simulink model "simAttitudeControl"  (R2014b)
settings: Solver=ode45  StartTime=0.0  StopTime=tof  FixedStep=dt  MaxStep=dtmax  RelTol=1e-3
values from neighbouring files (symbols this model uses):
  dtFc = 10e-3    (= 0.01)    [quadrotor.m]
  euler0 = [0 0 0]'*pi/180    [quadrotor.m]
  IxxT = 2.7e-3    (= 0.0027)    [quadrotor.m]
  IyyT = IxxT    (= 0.0027)    [quadrotor.m]
  IzzT = 5.2e-3    (= 0.0052)    [quadrotor.m]
  Kp = 2*0.75*diag([1 1 1])    [quadrotor.m]
  Kv = 0*0.005*diag([1 1 1])    [quadrotor.m]
  pqr0 = [0 0 0]'*pi/180    [quadrotor.m]
  q0 = [euler0 ; pqr0]    [quadrotor.m]
  Vb0 = [0 0 0]'    [quadrotor.m]
  Xe0 = [0 0 0]'    [quadrotor.m]
libraries: aerolibutil x10
settings Model: Creator=alp.marangoz  LastModifiedBy=alpmarangoz
settings SolverCC: AutoInsertRateTranBlk=on
settings DataIOCC: SignalLoggingSaveFormat=ModelDataLogs
settings OptimizationCC: ExpressionDepthLimit=2147483647
settings DebuggingCC: UnderspecifiedInitializationDetection=Classic  MergeDetectMultiDrivingBlocksExec=none  InheritedTsInSrcMsg=none  CheckMatrixSingularityMsg=error  FcnCallInpInsideContextMsg=UseLocalSettings  StateNameClashWarn=warning
settings GRTTargetCC: CombineOutputUpdateFcns=off  GRTInterface=on

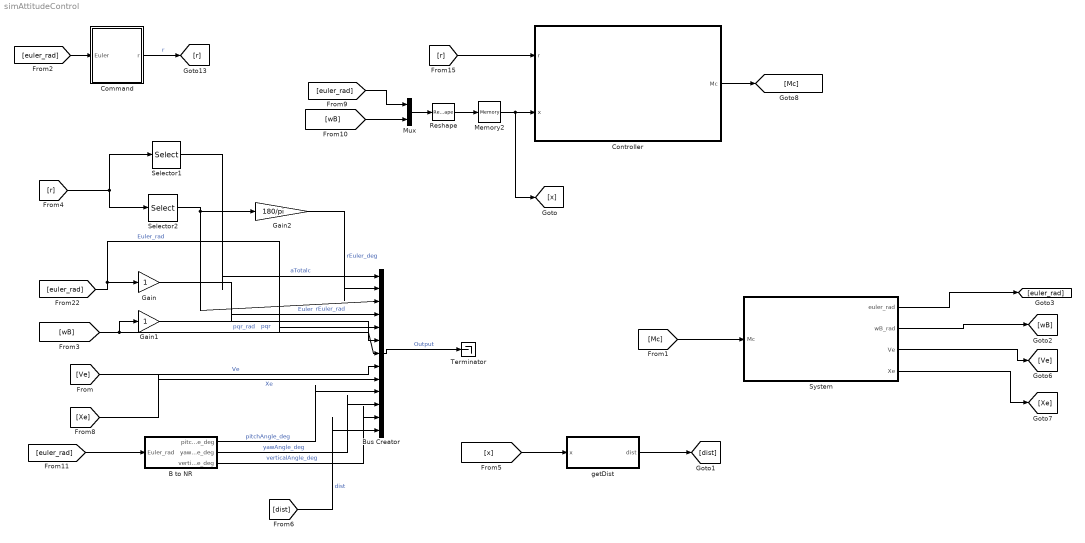
== system simAttitudeControl ==
  B to NR : Subsystem  TreatAsAtomicUnit=on
  Bus Creator : BusCreator  Inputs=13
  Command : Subsystem  TreatAsAtomicUnit=on  SystemSampleTime=dtFc
  Controller : Subsystem  TreatAsAtomicUnit=on  SystemSampleTime=dtFc
  Gain : Gain
  Gain1 : Gain
  Gain2 : Gain  Gain=180/pi
  Memory2 : Memory  X0=q0  InheritSampleTime=on  LinearizeMemory=on  LinearizeAsDelay=on
  Mux : Mux  Inputs=2
  Reshape : Reshape  OutputDimensionality=Column vector (2-D)
  Selector1 : Selector  NumberOfDimensions=2  InputPortWidth=2  IndexOptions=Index vector (dialog),Index vector (dialog)  Indices=1,1  OutputSizes=1,1
  Selector2 : Selector  NumberOfDimensions=2  InputPortWidth=3  IndexOptions=Index vector (dialog),Index vector (dialog)  Indices=[2 3 4],1  OutputSizes=1,1
  System : Subsystem  TreatAsAtomicUnit=on
  Terminator : Terminator
  getDist : Subsystem  TreatAsAtomicUnit=on
  wires:
  Command/1(r) -> [r]  "r"
  Controller/1(Mc) -> [Mc]
  [Mc] -> System/1(Mc)
  Reshape/1 -> Memory2/1
  [euler_rad] -> Command/1(Euler)
  Memory2/1 -> [x], Controller/2(x)
  [r] -> Controller/1(r)
  Bus Creator/1 -> Terminator/1  "Output"
  [r] -> Selector1/1, Selector2/1
  System/3(Ve) -> [Ve]
  System/4(Xe) -> [Xe]
  Selector1/1 -> Bus Creator/1  "aTotalc"
  Selector2/1 -> Gain2/1, Bus Creator/3  "rEuler_rad"
  [euler_rad] -> Gain/1, Bus Creator/5  "Euler_rad"
  [Ve] -> Bus Creator/8  "Ve"
  [Xe] -> Bus Creator/9  "Xe"
  System/1(euler_rad) -> [euler_rad]
  System/2(wB_rad) -> [wB]
  Mux/1 -> Reshape/1
  [euler_rad] -> Mux/1
  [wB] -> Mux/2
  Gain/1 -> Bus Creator/4  "Euler"
  [wB] -> Bus Creator/7, Gain1/1  "pqr_rad"
  Gain1/1 -> Bus Creator/6  "pqr"
  [euler_rad] -> B to NR/1(Euler_rad)
  B to NR/1(pitchAngle_deg) -> Bus Creator/10  "pitchAngle_deg"
  B to NR/2(yawAngle_deg) -> Bus Creator/11  "yawAngle_deg"
  B to NR/3(verticalAngle_deg) -> Bus Creator/12  "verticalAngle_deg"
  Gain2/1 -> Bus Creator/2  "rEuler_deg"
  [x] -> getDist/1(x)
  getDist/1(dist) -> [dist]
  [dist] -> Bus Creator/13  "dist"

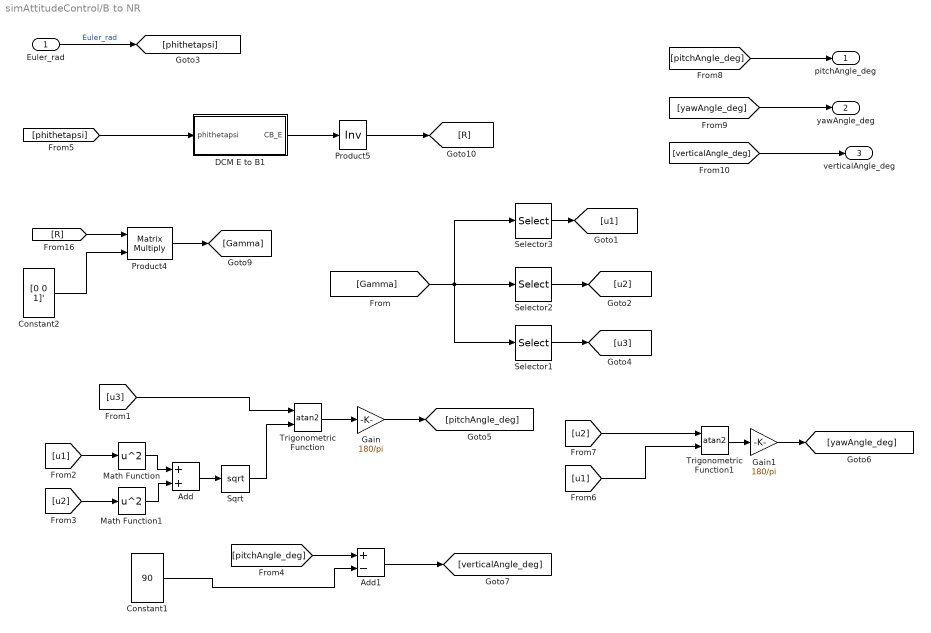
== system simAttitudeControl/B to NR ==
  Euler_rad : Inport
  Add : Sum
  Add1 : Sum  Inputs=+-
  Constant1 : Constant  Value=90  VectorParams1D=off
  Constant2 : Constant  Value=[0 0 1]'  VectorParams1D=off
  DCM E to B1 : Subsystem
  Gain : Gain  Gain=180/pi
  Gain1 : Gain  Gain=180/pi
  Math Function : Math  Operator=square  SaturateOnIntegerOverflow=on
  Math Function1 : Math  Operator=square  SaturateOnIntegerOverflow=on
  Product4 : Product  Multiplication=Matrix(*)  RndMeth=Zero
  Product5 : Product  Inputs=/  Multiplication=Matrix(*)  RndMeth=Zero
  Selector1 : Selector  InputPortWidth=3  Indices=3
  Selector2 : Selector  InputPortWidth=3  Indices=2
  Selector3 : Selector  InputPortWidth=3
  Sqrt : Sqrt  SaturateOnIntegerOverflow=on
  Trigonometric Function : Trigonometry  Operator=atan2
  Trigonometric Function1 : Trigonometry  Operator=atan2
  pitchAngle_deg : Outport
  yawAngle_deg : Outport  Port=2
  verticalAngle_deg : Outport  Port=3
  wires:
  Euler_rad/1 -> [phithetapsi]  "Euler_rad"
  Product5/1 -> [R]
  [phithetapsi] -> DCM E to B1/1(phithetapsi)
  DCM E to B1/1(CB_E) -> Product5/1
  [R] -> Product4/1
  Constant2/1 -> Product4/2
  Product4/1 -> [Gamma]
  [Gamma] -> Selector1/1, Selector3/1, Selector2/1
  Selector3/1 -> [u1]
  Selector2/1 -> [u2]
  Selector1/1 -> [u3]
  [u1] -> Math Function/1
  [u2] -> Math Function1/1
  Math Function/1 -> Add/1
  Math Function1/1 -> Add/2
  Add/1 -> Sqrt/1
  [u3] -> Trigonometric Function/1
  Sqrt/1 -> Trigonometric Function/2
  Trigonometric Function/1 -> Gain/1
  Trigonometric Function1/1 -> Gain1/1
  [u2] -> Trigonometric Function1/1
  [u1] -> Trigonometric Function1/2
  [yawAngle_deg] -> yawAngle_deg/1
  [pitchAngle_deg] -> pitchAngle_deg/1
  Gain/1 -> [pitchAngle_deg]
  Gain1/1 -> [yawAngle_deg]
  Constant1/1 -> Add1/2
  [pitchAngle_deg] -> Add1/1
  Add1/1 -> [verticalAngle_deg]
  [verticalAngle_deg] -> verticalAngle_deg/1

== system simAttitudeControl/Command ==
  Euler : Inport
  From Workspace : FromWorkspace  VariableName=r  Interpolate=off  OutputAfterFinalValue=Setting to zero
  Memory2 : Memory  X0=euler0  InheritSampleTime=on  LinearizeMemory=on  LinearizeAsDelay=on
  Reshape1 : Reshape  OutputDimensionality=Column vector (2-D)
  Selector : Selector  NumberOfDimensions=2  InputPortWidth=2  IndexOptions=Index vector (dialog),Index vector (dialog)  Indices=1,1  OutputSizes=1,1
  Selector1 : Selector  NumberOfDimensions=2  InputPortWidth=3  IndexOptions=Index vector (dialog),Index vector (dialog)  Indices=[2 3 4],1  OutputSizes=1,1
  Subtract : Sum  Inputs=+-
  Terminator : Terminator
  Terminator1 : Terminator
  Terminator2 : Terminator
  r : Outport  InitialOutput=0
  wires:
  From Workspace/1 -> Reshape1/1
  Reshape1/1 -> r/1, Selector/1, Selector1/1
  Euler/1 -> Memory2/1
  Memory2/1 -> [euler]
  [euler] -> Subtract/2  "q"
  Selector/1 -> Terminator/1  "rnc"
  Selector1/1 -> Terminator2/1, Subtract/1  "rEuler"
  Subtract/1 -> Terminator1/1  "eEuler"

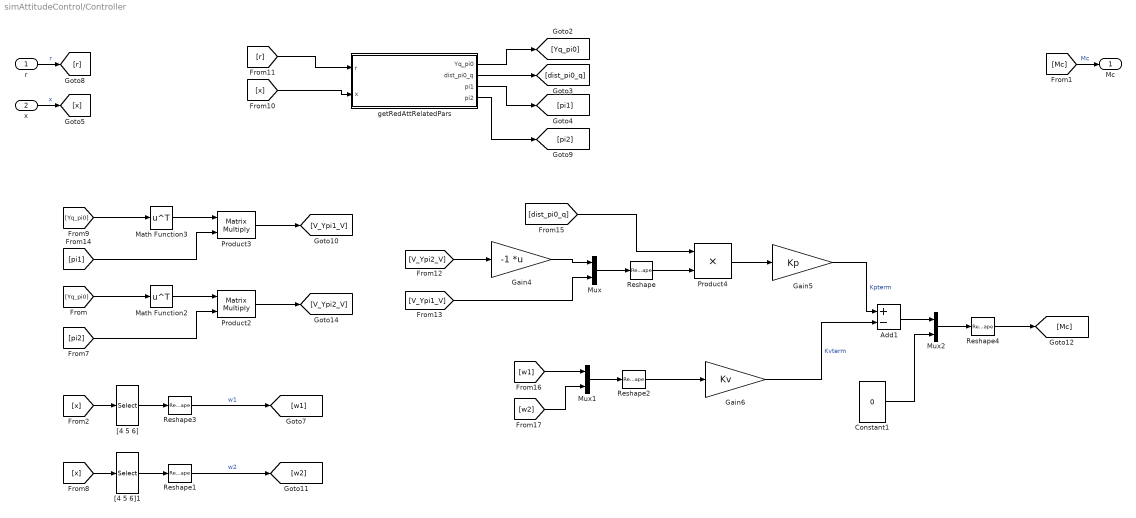
== system simAttitudeControl/Controller ==
  r : Inport
  x : Inport  Port=2
  Add1 : Sum  Inputs=+-
  Constant1 : Constant  Value=0  VectorParams1D=off
  Gain4 : Gain  Gain=-1  Multiplication=Matrix(K*u)
  Gain5 : Gain  Gain=Kp
  Gain6 : Gain  Gain=Kv
  Math Function2 : Math  Operator=transpose  SaturateOnIntegerOverflow=on
  Math Function3 : Math  Operator=transpose  SaturateOnIntegerOverflow=on
  Mux : Mux  Inputs=2
  Mux1 : Mux  Inputs=2
  Mux2 : Mux  Inputs=2
  Product2 : Product  Multiplication=Matrix(*)  RndMeth=Zero
  Product3 : Product  Multiplication=Matrix(*)  RndMeth=Zero
  Product4 : Product  RndMeth=Zero
  Reshape{,1..4} (5 alike) : Reshape  OutputDimensionality=Column vector (2-D)
  "[4 5 6]" : Selector  InputPortWidth=6  Indices=4
  "[4 5 6]1" : Selector  InputPortWidth=6  Indices=5
  getRedAttRelatedPars : Subsystem
  Mc : Outport
  wires:
  r/1 -> [r]  "r"
  x/1 -> [x]  "x"
  [Mc] -> Mc/1  "Mc"
  [x] -> getRedAttRelatedPars/2(x)
  [r] -> getRedAttRelatedPars/1(r)
  getRedAttRelatedPars/2(dist_pi0_q) -> [dist_pi0_q]
  getRedAttRelatedPars/1(Yq_pi0) -> [Yq_pi0]
  getRedAttRelatedPars/3(pi1) -> [pi1]
  getRedAttRelatedPars/4(pi2) -> [pi2]
  [Yq_pi0] -> Math Function2/1
  Math Function2/1 -> Product2/1
  [pi2] -> Product2/2
  Product2/1 -> [V_Ypi2_V]
  [Yq_pi0] -> Math Function3/1
  Math Function3/1 -> Product3/1
  [pi1] -> Product3/2
  Product3/1 -> [V_Ypi1_V]
  Reshape3/1 -> [w1]  "w1"
  "[4 5 6]"/1 -> Reshape3/1
  [x] -> "[4 5 6]"/1
  Reshape1/1 -> [w2]  "w2"
  "[4 5 6]1"/1 -> Reshape1/1
  [x] -> "[4 5 6]1"/1
  [V_Ypi2_V] -> Gain4/1
  Gain4/1 -> Mux/1
  [V_Ypi1_V] -> Mux/2
  Mux/1 -> Reshape/1
  [dist_pi0_q] -> Product4/1
  Reshape/1 -> Product4/2
  Product4/1 -> Gain5/1
  Mux1/1 -> Reshape2/1
  [w1] -> Mux1/1
  [w2] -> Mux1/2
  Reshape2/1 -> Gain6/1
  Gain5/1 -> Add1/1  "Kpterm"
  Gain6/1 -> Add1/2  "Kvterm"
  Mux2/1 -> Reshape4/1
  Add1/1 -> Mux2/1
  Constant1/1 -> Mux2/2
  Reshape4/1 -> [Mc]

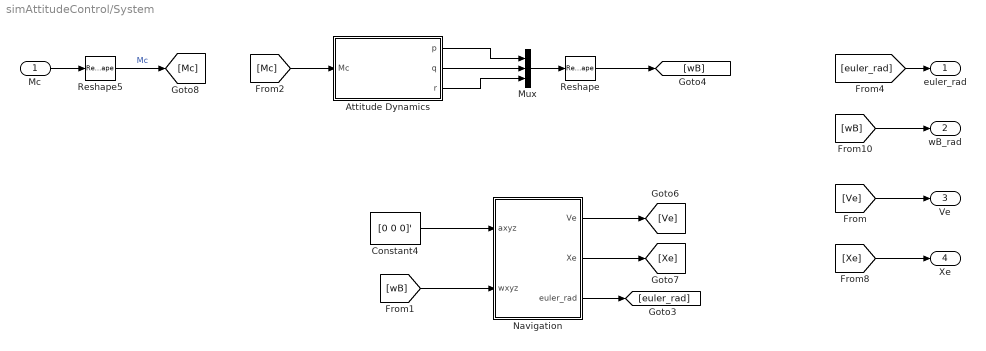
== system simAttitudeControl/System ==
  Mc : Inport
  Attitude Dynamics : Subsystem
  Constant4 : Constant  Value=[0 0 0]'  VectorParams1D=off
  Mux : Mux  Inputs=3
  Navigation : Subsystem
  Reshape : Reshape  OutputDimensionality=Column vector (2-D)
  Reshape5 : Reshape  OutputDimensionality=Column vector (2-D)
  euler_rad : Outport
  wB_rad : Outport  Port=2
  Ve : Outport  Port=3
  Xe : Outport  Port=4
  wires:
  Mc/1 -> Reshape5/1
  Reshape5/1 -> [Mc]  "Mc"
  [euler_rad] -> euler_rad/1
  Constant4/1 -> Navigation/1(axyz)
  [wB] -> Navigation/2(wxyz)
  Navigation/1(Ve) -> [Ve]
  Navigation/2(Xe) -> [Xe]
  Navigation/3(euler_rad) -> [euler_rad]
  [Xe] -> Xe/1
  [Ve] -> Ve/1
  [wB] -> wB_rad/1
  Attitude Dynamics/1(p) -> Mux/1
  Attitude Dynamics/2(q) -> Mux/2
  Attitude Dynamics/3(r) -> Mux/3
  Mux/1 -> Reshape/1
  Reshape/1 -> [wB]
  [Mc] -> Attitude Dynamics/1(Mc)

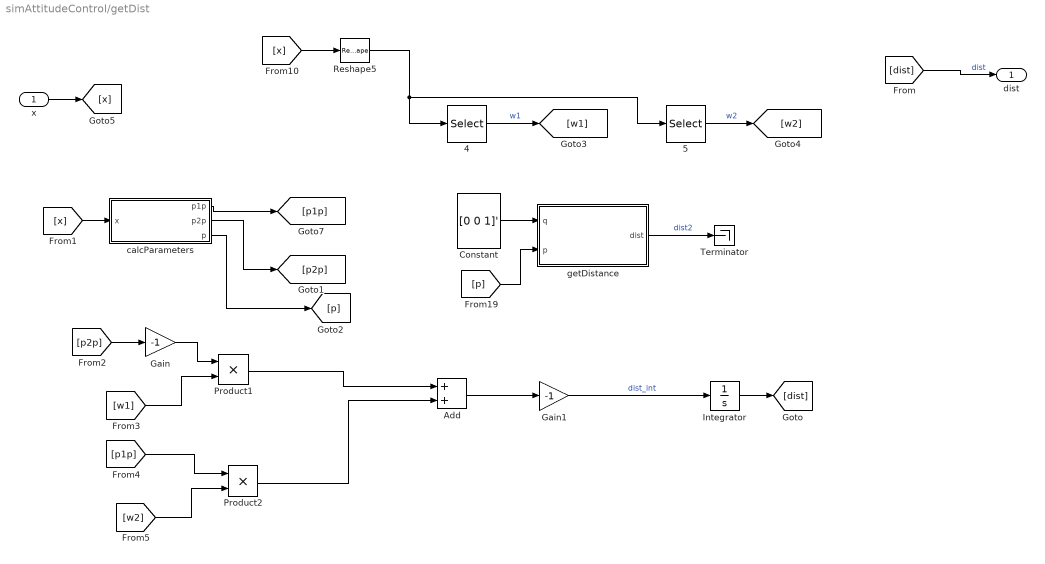
== system simAttitudeControl/getDist ==
  x : Inport
  4 : Selector  NumberOfDimensions=2  InputPortWidth=3  IndexOptions=Index vector (dialog),Index vector (dialog)  Indices=4,1  OutputSizes=1,1
  5 : Selector  NumberOfDimensions=2  InputPortWidth=3  IndexOptions=Index vector (dialog),Index vector (dialog)  Indices=5,1  OutputSizes=1,1
  Add : Sum
  Constant : Constant  Value=[0 0 1]'  VectorParams1D=off
  Gain : Gain  Gain=-1
  Gain1 : Gain  Gain=-1
  Integrator : Integrator
  Product1 : Product
  Product2 : Product
  Reshape5 : Reshape  OutputDimensionality=Column vector (2-D)
  Terminator : Terminator
  calcParameters : Subsystem  TreatAsAtomicUnit=on
  getDistance : Subsystem
  dist : Outport
  wires:
  x/1 -> [x]
  Reshape5/1 -> 5/1, 4/1
  [x] -> Reshape5/1
  [dist] -> dist/1  "dist"
  [x] -> calcParameters/1(x)
  calcParameters/1(p1p) -> [p1p]
  calcParameters/2(p2p) -> [p2p]
  4/1 -> [w1]  "w1"
  5/1 -> [w2]  "w2"
  [w1] -> Product1/2
  [p1p] -> Product2/1
  [w2] -> Product2/2
  [p2p] -> Gain/1
  Gain/1 -> Product1/1
  Product1/1 -> Add/1
  Product2/1 -> Add/2
  Add/1 -> Gain1/1
  Gain1/1 -> Integrator/1  "dist_int"
  Integrator/1 -> [dist]
  getDistance/1(dist) -> Terminator/1  "dist2"
  Constant/1 -> getDistance/1(q)
  [p] -> getDistance/2(p)
  calcParameters/3(p) -> [p]

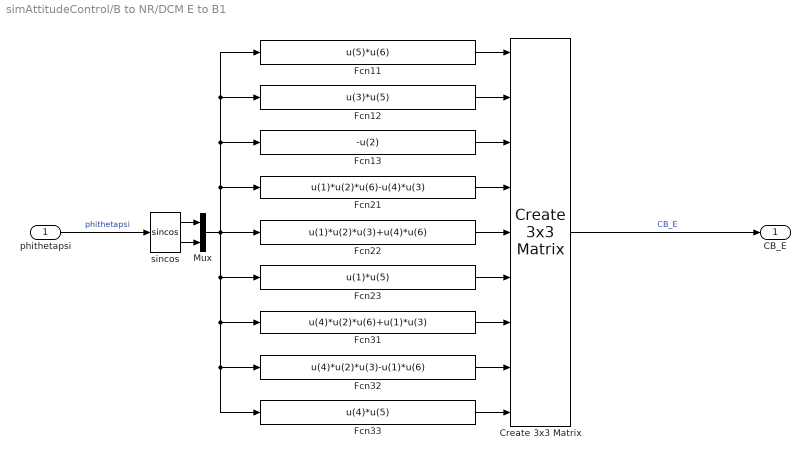
== system simAttitudeControl/B to NR/DCM E to B1 ==
  phithetapsi : Inport
  Create 3x3 Matrix : aerolibutil/Create 3x3 Matrix
  Fcn11 : Fcn  Expr=u(5)*u(6)
  Fcn12 : Fcn  Expr=u(3)*u(5)
  Fcn13 : Fcn  Expr=-u(2)
  Fcn21 : Fcn  Expr=u(1)*u(2)*u(6)-u(4)*u(3)
  Fcn22 : Fcn  Expr=u(1)*u(2)*u(3)+u(4)*u(6)
  Fcn23 : Fcn  Expr=u(1)*u(5)
  Fcn31 : Fcn  Expr=u(4)*u(2)*u(6)+u(1)*u(3)
  Fcn32 : Fcn  Expr=u(4)*u(2)*u(3)-u(1)*u(6)
  Fcn33 : Fcn  Expr=u(4)*u(5)
  Mux : Mux  Inputs=2
  sincos : Trigonometry  Operator=sincos
  CB_E : Outport
  wires:
  Create 3x3 Matrix/1 -> CB_E/1  "CB_E"
  phithetapsi/1 -> sincos/1  "phithetapsi"
  Fcn33/1 -> Create 3x3 Matrix/9
  Fcn32/1 -> Create 3x3 Matrix/8
  Fcn23/1 -> Create 3x3 Matrix/6
  Fcn22/1 -> Create 3x3 Matrix/5
  Fcn31/1 -> Create 3x3 Matrix/7
  Fcn21/1 -> Create 3x3 Matrix/4
  Fcn13/1 -> Create 3x3 Matrix/3
  Fcn12/1 -> Create 3x3 Matrix/2
  Fcn11/1 -> Create 3x3 Matrix/1
  Mux/1 -> Fcn21/1, Fcn13/1, Fcn12/1, Fcn11/1, Fcn22/1, Fcn23/1, Fcn31/1, Fcn33/1, Fcn32/1
  sincos/2 -> Mux/2
  sincos/1 -> Mux/1

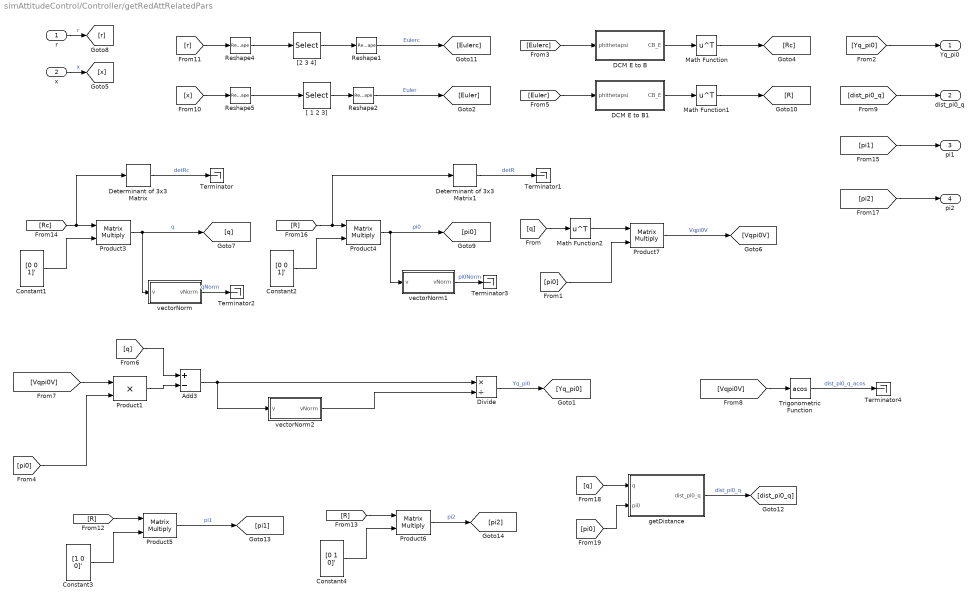
== system simAttitudeControl/Controller/getRedAttRelatedPars ==
  r : Inport
  x : Inport  Port=2
  Add3 : Sum  Inputs=+-
  Constant1 : Constant  Value=[0 0 1]'  VectorParams1D=off
  Constant2 : Constant  Value=[0 0 1]'  VectorParams1D=off
  Constant3 : Constant  Value=[1 0 0]'  VectorParams1D=off
  Constant4 : Constant  Value=[0 1 0]'  VectorParams1D=off
  DCM E to B : Subsystem
  DCM E to B1 : Subsystem
  Determinant of 3x3 Matrix : aerolibutil/Determinant of 3x3 Matrix
  Determinant of 3x3 Matrix1 : aerolibutil/Determinant of 3x3 Matrix
  Divide : Product  Inputs=*/
  Math Function : Math  Operator=transpose  SaturateOnIntegerOverflow=on
  Math Function1 : Math  Operator=transpose  SaturateOnIntegerOverflow=on
  Math Function2 : Math  Operator=transpose  SaturateOnIntegerOverflow=on
  Product1 : Product  RndMeth=Zero
  Product{3..7} (5 alike) : Product  Multiplication=Matrix(*)  RndMeth=Zero
  Reshape{1..2,4..5} (4 alike) : Reshape  OutputDimensionality=Column vector (2-D)
  Terminator{,1..4} (5 alike) : Terminator
  Trigonometric Function : Trigonometry  Operator=acos
  "[ 1 2 3]" : Selector  NumberOfDimensions=2  InputPortWidth=3  IndexOptions=Index vector (dialog),Index vector (dialog)  Indices=[1 2 3],1  OutputSizes=1,1
  "[2 3 4]" : Selector  NumberOfDimensions=2  InputPortWidth=3  IndexOptions=Index vector (dialog),Index vector (dialog)  Indices=[2 3 4],1  OutputSizes=1,1
  getDistance : Subsystem
  vectorNorm : Subsystem
  vectorNorm1 : Subsystem
  vectorNorm2 : Subsystem
  Yq_pi0 : Outport
  dist_pi0_q : Outport  Port=2
  pi1 : Outport  Port=3
  pi2 : Outport  Port=4
  wires:
  DCM E to B1/1(CB_E) -> Math Function1/1
  [Euler] -> DCM E to B1/1(phithetapsi)
  Reshape4/1 -> "[2 3 4]"/1
  DCM E to B/1(CB_E) -> Math Function/1
  [Eulerc] -> DCM E to B/1(phithetapsi)
  [r] -> Reshape4/1
  "[2 3 4]"/1 -> Reshape1/1
  Reshape1/1 -> [Eulerc]  "Eulerc"
  Reshape2/1 -> [Euler]  "Euler"
  Reshape5/1 -> "[ 1 2 3]"/1
  "[ 1 2 3]"/1 -> Reshape2/1
  Math Function/1 -> [Rc]
  [x] -> Reshape5/1
  Math Function1/1 -> [R]
  x/1 -> [x]  "x"
  r/1 -> [r]  "r"
  Product4/1 -> vectorNorm1/1(v), [pi0]  "pi0"
  Constant2/1 -> Product4/2
  [R] -> Determinant of 3x3 Matrix1/1, Product4/1
  Product3/1 -> vectorNorm/1(v), [q]  "q"
  Constant1/1 -> Product3/2
  [Rc] -> Determinant of 3x3 Matrix/1, Product3/1
  [dist_pi0_q] -> dist_pi0_q/1
  [q] -> Math Function2/1
  Math Function2/1 -> Product7/1
  [pi0] -> Product7/2
  [pi0] -> Product1/2
  [q] -> Add3/1
  Product1/1 -> Add3/2
  Add3/1 -> vectorNorm2/1(v), Divide/1
  vectorNorm2/1(vNorm) -> Divide/2
  Divide/1 -> [Yq_pi0]  "Yq_pi0"
  Product7/1 -> [Vqpi0V]  "Vqpi0V"
  [Vqpi0V] -> Product1/1
  [Vqpi0V] -> Trigonometric Function/1
  Trigonometric Function/1 -> Terminator4/1  "dist_pi0_q_acos"
  [Yq_pi0] -> Yq_pi0/1
  Product5/1 -> [pi1]  "pi1"
  Constant3/1 -> Product5/2
  [R] -> Product5/1
  Product6/1 -> [pi2]  "pi2"
  Constant4/1 -> Product6/2
  [R] -> Product6/1
  [pi1] -> pi1/1
  [pi2] -> pi2/1
  Determinant of 3x3 Matrix/1 -> Terminator/1  "detRc"
  Determinant of 3x3 Matrix1/1 -> Terminator1/1  "detR"
  vectorNorm/1(vNorm) -> Terminator2/1  "qNorm"
  vectorNorm1/1(vNorm) -> Terminator3/1  "pi0Norm"
  getDistance/1(dist_pi0_q) -> [dist_pi0_q]  "dist_pi0_q"
  [q] -> getDistance/1(q)
  [pi0] -> getDistance/2(pi0)

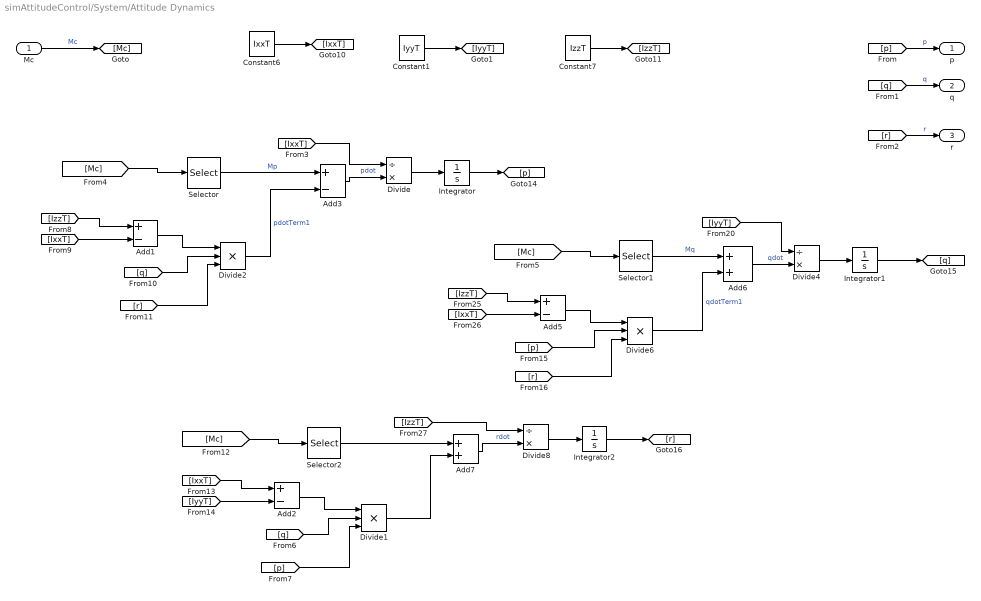
== system simAttitudeControl/System/Attitude Dynamics ==
  Mc : Inport
  Add{1..3,5} (4 alike) : Sum  Inputs=+-
  Add6 : Sum
  Add7 : Sum
  Constant1 : Constant  Value=IyyT  VectorParams1D=off
  Constant6 : Constant  Value=IxxT  VectorParams1D=off
  Constant7 : Constant  Value=IzzT  VectorParams1D=off
  Divide : Product  Inputs=/*
  Divide1 : Product  Inputs=***
  Divide2 : Product  Inputs=***
  Divide4 : Product  Inputs=/*
  Divide6 : Product  Inputs=***
  Divide8 : Product  Inputs=/*
  Integrator : Integrator  InitialCondition=pqr0(1)
  Integrator1 : Integrator  InitialCondition=pqr0(2)
  Integrator2 : Integrator  InitialCondition=pqr0(3)
  Selector : Selector  InputPortWidth=3  Indices=[1]
  Selector1 : Selector  InputPortWidth=3  Indices=[2]
  Selector2 : Selector  InputPortWidth=3  Indices=[3]
  p : Outport
  q : Outport  Port=2
  r : Outport  Port=3
  wires:
  Mc/1 -> [Mc]  "Mc"
  Constant6/1 -> [IxxT]
  Constant7/1 -> [IzzT]
  [p] -> p/1  "p"
  [q] -> q/1  "q"
  [r] -> r/1  "r"
  Integrator/1 -> [p]
  Divide/1 -> Integrator/1
  [IxxT] -> Divide/1
  [IzzT] -> Add1/1
  [IxxT] -> Add1/2
  Add1/1 -> Divide2/1
  [q] -> Divide2/2
  [r] -> Divide2/3
  Add3/1 -> Divide/2  "pdot"
  Selector/1 -> Add3/1  "Mp"
  Divide2/1 -> Add3/2  "pdotTerm1"
  Integrator1/1 -> [q]
  Divide4/1 -> Integrator1/1
  [IyyT] -> Divide4/1
  [IzzT] -> Add5/1
  [IxxT] -> Add5/2
  Add5/1 -> Divide6/1
  [p] -> Divide6/2
  Add6/1 -> Divide4/2  "qdot"
  Divide6/1 -> Add6/2  "qdotTerm1"
  Integrator2/1 -> [r]
  Divide8/1 -> Integrator2/1
  [IzzT] -> Divide8/1
  Add7/1 -> Divide8/2  "rdot"
  [Mc] -> Selector/1
  Selector1/1 -> Add6/1  "Mq"
  [Mc] -> Selector1/1
  [IxxT] -> Add2/1
  [IyyT] -> Add2/2
  Add2/1 -> Divide1/1
  [q] -> Divide1/2
  [p] -> Divide1/3
  [Mc] -> Selector2/1
  Selector2/1 -> Add7/1
  Divide1/1 -> Add7/2
  Constant1/1 -> [IyyT]
  [r] -> Divide6/3

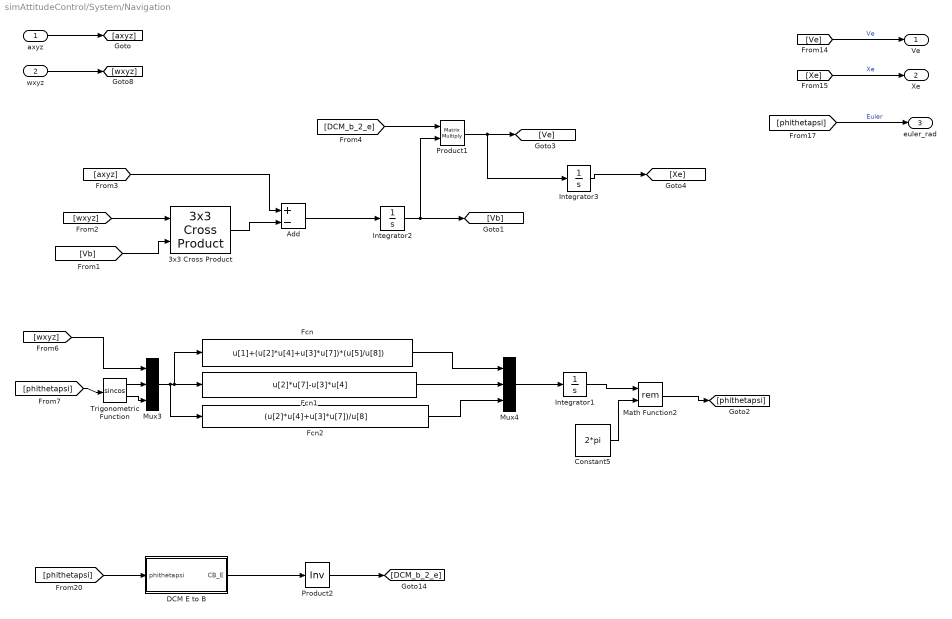
== system simAttitudeControl/System/Navigation ==
  axyz : Inport
  wxyz : Inport  Port=2
  3x3 Cross Product : aerolibutil/3x3 Cross Product
  Add : Sum  Inputs=+-
  Constant5 : Constant  Value=2*pi
  DCM E to B : Subsystem
  Fcn : Fcn  Expr=u[1]+(u[2]*u[4]+u[3]*u[7])*(u[5]/u[8])
  Fcn1 : Fcn  Expr=u[2]*u[7]-u[3]*u[4]
  Fcn2 : Fcn  Expr=(u[2]*u[4]+u[3]*u[7])/u[8]
  Integrator1 : Integrator  InitialCondition=euler0
  Integrator2 : Integrator  InitialCondition=Vb0
  Integrator3 : Integrator  InitialCondition=Xe0
  Math Function2 : Math  Operator=rem  SaturateOnIntegerOverflow=on
  Mux3 : Mux  Inputs=3
  Mux4 : Mux  Inputs=3
  Product1 : Product  Multiplication=Matrix(*)  RndMeth=Zero
  Product2 : Product  Inputs=/  Multiplication=Matrix(*)  RndMeth=Zero
  Trigonometric Function : Trigonometry  Operator=sincos
  Ve : Outport
  Xe : Outport  Port=2
  euler_rad : Outport  Port=3
  wires:
  axyz/1 -> [axyz]
  wxyz/1 -> [wxyz]
  [phithetapsi] -> euler_rad/1  "Euler"
  [Ve] -> Ve/1  "Ve"
  [Xe] -> Xe/1  "Xe"
  [wxyz] -> Mux3/1
  Trigonometric Function/1 -> Mux3/2
  Trigonometric Function/2 -> Mux3/3
  [phithetapsi] -> Trigonometric Function/1
  Mux3/1 -> Fcn1/1, Fcn/1, Fcn2/1
  Fcn/1 -> Mux4/1
  Fcn1/1 -> Mux4/2
  Fcn2/1 -> Mux4/3
  Mux4/1 -> Integrator1/1
  Integrator1/1 -> Math Function2/1
  Constant5/1 -> Math Function2/2
  Math Function2/1 -> [phithetapsi]
  [wxyz] -> 3x3 Cross Product/1
  [Vb] -> 3x3 Cross Product/2
  [axyz] -> Add/1
  3x3 Cross Product/1 -> Add/2
  Add/1 -> Integrator2/1
  Integrator2/1 -> [Vb], Product1/2
  [DCM_b_2_e] -> Product1/1
  Product1/1 -> [Ve], Integrator3/1
  Integrator3/1 -> [Xe]
  [phithetapsi] -> DCM E to B/1(phithetapsi)
  DCM E to B/1(CB_E) -> Product2/1
  Product2/1 -> [DCM_b_2_e]

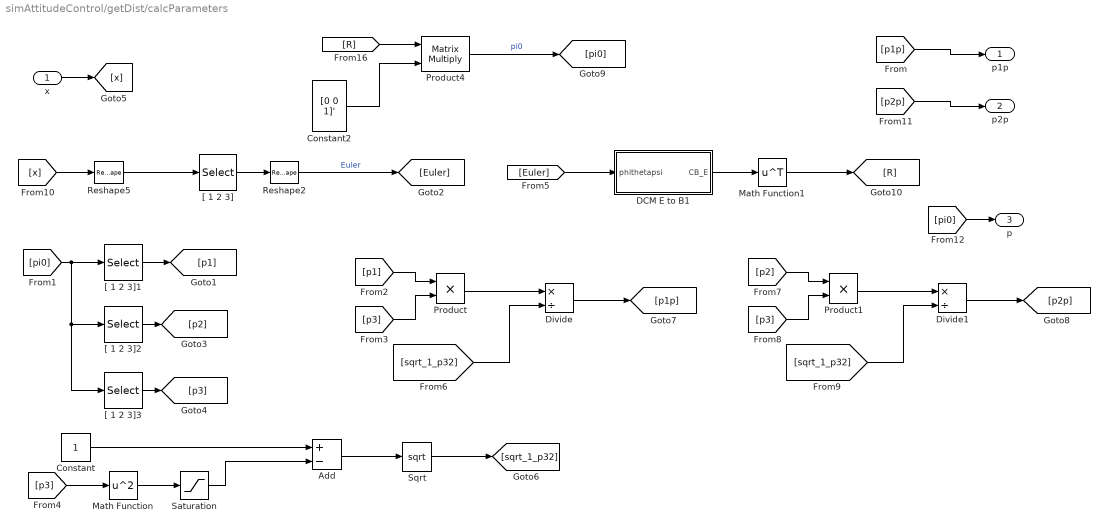
== system simAttitudeControl/getDist/calcParameters ==
  x : Inport
  Add : Sum  Inputs=+-
  Constant : Constant
  Constant2 : Constant  Value=[0 0 1]'  VectorParams1D=off
  DCM E to B1 : Subsystem
  Divide : Product  Inputs=*/
  Divide1 : Product  Inputs=*/
  Math Function : Math  Operator=square  SaturateOnIntegerOverflow=on
  Math Function1 : Math  Operator=transpose  SaturateOnIntegerOverflow=on
  Product : Product
  Product1 : Product
  Product4 : Product  Multiplication=Matrix(*)  RndMeth=Zero
  Reshape2 : Reshape  OutputDimensionality=Column vector (2-D)
  Reshape5 : Reshape  OutputDimensionality=Column vector (2-D)
  Saturation : Saturate  UpperLimit=0.999999  LowerLimit=0
  Sqrt : Sqrt  SaturateOnIntegerOverflow=on
  "[ 1 2 3]" : Selector  NumberOfDimensions=2  InputPortWidth=3  IndexOptions=Index vector (dialog),Index vector (dialog)  Indices=[1 2 3],1  OutputSizes=1,1
  "[ 1 2 3]1" : Selector  InputPortWidth=3
  "[ 1 2 3]2" : Selector  InputPortWidth=3  Indices=2
  "[ 1 2 3]3" : Selector  InputPortWidth=3  Indices=3
  p1p : Outport
  p2p : Outport  Port=2
  p : Outport  Port=3
  wires:
  [sqrt_1_p32] -> Divide1/2
  Product1/1 -> Divide1/1
  Divide1/1 -> [p2p]
  [p3] -> Product1/2
  [p2] -> Product1/1
  [sqrt_1_p32] -> Divide/2
  Product/1 -> Divide/1
  Divide/1 -> [p1p]
  Sqrt/1 -> [sqrt_1_p32]
  [p3] -> Math Function/1
  Constant/1 -> Add/1
  Math Function/1 -> Saturation/1
  Add/1 -> Sqrt/1
  [p3] -> Product/2
  [p1] -> Product/1
  "[ 1 2 3]3"/1 -> [p3]
  "[ 1 2 3]2"/1 -> [p2]
  "[ 1 2 3]1"/1 -> [p1]
  [pi0] -> "[ 1 2 3]1"/1, "[ 1 2 3]2"/1, "[ 1 2 3]3"/1
  [p1p] -> p1p/1
  [R] -> Product4/1
  Constant2/1 -> Product4/2
  Product4/1 -> [pi0]  "pi0"
  Math Function1/1 -> [R]
  [x] -> Reshape5/1
  "[ 1 2 3]"/1 -> Reshape2/1
  Reshape5/1 -> "[ 1 2 3]"/1
  Reshape2/1 -> [Euler]  "Euler"
  [Euler] -> DCM E to B1/1(phithetapsi)
  DCM E to B1/1(CB_E) -> Math Function1/1
  x/1 -> [x]
  [p2p] -> p2p/1
  Saturation/1 -> Add/2
  [pi0] -> p/1

== system simAttitudeControl/getDist/getDistance ==
  q : Inport
  p : Inport  Port=2
  3x3 Cross Product1 : aerolibutil/3x3 Cross Product
  Trigonometric Function : Trigonometry  Operator=asin
  vectorNorm : Subsystem
  dist : Outport
  wires:
  [q] -> 3x3 Cross Product1/2
  [pi0] -> 3x3 Cross Product1/1
  3x3 Cross Product1/1 -> vectorNorm/1(v)
  [dist_pi0_q] -> dist/1
  p/1 -> [pi0]
  q/1 -> [q]
  Trigonometric Function/1 -> [dist_pi0_q]
  vectorNorm/1(vNorm) -> Trigonometric Function/1

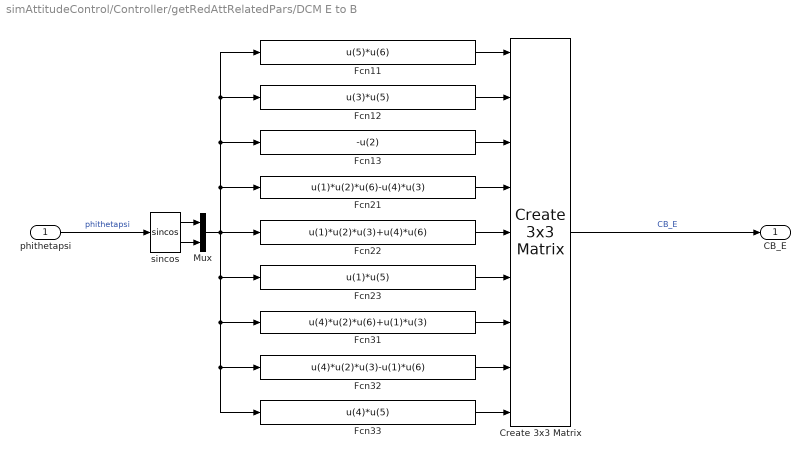
== system simAttitudeControl/Controller/getRedAttRelatedPars/DCM E to B ==
  phithetapsi : Inport
  Create 3x3 Matrix : aerolibutil/Create 3x3 Matrix
  Fcn11 : Fcn  Expr=u(5)*u(6)
  Fcn12 : Fcn  Expr=u(3)*u(5)
  Fcn13 : Fcn  Expr=-u(2)
  Fcn21 : Fcn  Expr=u(1)*u(2)*u(6)-u(4)*u(3)
  Fcn22 : Fcn  Expr=u(1)*u(2)*u(3)+u(4)*u(6)
  Fcn23 : Fcn  Expr=u(1)*u(5)
  Fcn31 : Fcn  Expr=u(4)*u(2)*u(6)+u(1)*u(3)
  Fcn32 : Fcn  Expr=u(4)*u(2)*u(3)-u(1)*u(6)
  Fcn33 : Fcn  Expr=u(4)*u(5)
  Mux : Mux  Inputs=2
  sincos : Trigonometry  Operator=sincos
  CB_E : Outport
  wires:
  sincos/1 -> Mux/1
  sincos/2 -> Mux/2
  Mux/1 -> Fcn32/1, Fcn33/1, Fcn31/1, Fcn23/1, Fcn22/1, Fcn11/1, Fcn12/1, Fcn13/1, Fcn21/1
  Fcn11/1 -> Create 3x3 Matrix/1
  Fcn12/1 -> Create 3x3 Matrix/2
  Fcn13/1 -> Create 3x3 Matrix/3
  Fcn21/1 -> Create 3x3 Matrix/4
  Fcn31/1 -> Create 3x3 Matrix/7
  Fcn22/1 -> Create 3x3 Matrix/5
  Fcn23/1 -> Create 3x3 Matrix/6
  Fcn32/1 -> Create 3x3 Matrix/8
  Fcn33/1 -> Create 3x3 Matrix/9
  phithetapsi/1 -> sincos/1  "phithetapsi"
  Create 3x3 Matrix/1 -> CB_E/1  "CB_E"

== system simAttitudeControl/Controller/getRedAttRelatedPars/DCM E to B1 ==
  phithetapsi : Inport
  Create 3x3 Matrix : aerolibutil/Create 3x3 Matrix
  Fcn11 : Fcn  Expr=u(5)*u(6)
  Fcn12 : Fcn  Expr=u(3)*u(5)
  Fcn13 : Fcn  Expr=-u(2)
  Fcn21 : Fcn  Expr=u(1)*u(2)*u(6)-u(4)*u(3)
  Fcn22 : Fcn  Expr=u(1)*u(2)*u(3)+u(4)*u(6)
  Fcn23 : Fcn  Expr=u(1)*u(5)
  Fcn31 : Fcn  Expr=u(4)*u(2)*u(6)+u(1)*u(3)
  Fcn32 : Fcn  Expr=u(4)*u(2)*u(3)-u(1)*u(6)
  Fcn33 : Fcn  Expr=u(4)*u(5)
  Mux : Mux  Inputs=2
  sincos : Trigonometry  Operator=sincos
  CB_E : Outport
  wires:
  sincos/1 -> Mux/1
  sincos/2 -> Mux/2
  Mux/1 -> Fcn32/1, Fcn33/1, Fcn31/1, Fcn23/1, Fcn22/1, Fcn11/1, Fcn12/1, Fcn13/1, Fcn21/1
  Fcn11/1 -> Create 3x3 Matrix/1
  Fcn12/1 -> Create 3x3 Matrix/2
  Fcn13/1 -> Create 3x3 Matrix/3
  Fcn21/1 -> Create 3x3 Matrix/4
  Fcn31/1 -> Create 3x3 Matrix/7
  Fcn22/1 -> Create 3x3 Matrix/5
  Fcn23/1 -> Create 3x3 Matrix/6
  Fcn32/1 -> Create 3x3 Matrix/8
  Fcn33/1 -> Create 3x3 Matrix/9
  phithetapsi/1 -> sincos/1  "phithetapsi"
  Create 3x3 Matrix/1 -> CB_E/1  "CB_E"

== system simAttitudeControl/Controller/getRedAttRelatedPars/getDistance ==
  q : Inport
  pi0 : Inport  Port=2
  3x3 Cross Product1 : aerolibutil/3x3 Cross Product
  Trigonometric Function : Trigonometry  Operator=asin
  vectorNorm : Subsystem
  dist_pi0_q : Outport
  wires:
  [q] -> 3x3 Cross Product1/2
  [pi0] -> 3x3 Cross Product1/1
  3x3 Cross Product1/1 -> vectorNorm/1(v)
  [dist_pi0_q] -> dist_pi0_q/1
  pi0/1 -> [pi0]
  q/1 -> [q]
  Trigonometric Function/1 -> [dist_pi0_q]
  vectorNorm/1(vNorm) -> Trigonometric Function/1

== system simAttitudeControl/Controller/getRedAttRelatedPars/vectorNorm ==
  v : Inport
  Math Function4 : Math  Operator=transpose  SaturateOnIntegerOverflow=on
  Product8 : Product  Multiplication=Matrix(*)  RndMeth=Zero
  Sqrt1 : Sqrt  SaturateOnIntegerOverflow=on
  vNorm : Outport
  wires:
  Sqrt1/1 -> vNorm/1
  v/1 -> Product8/2, Math Function4/1
  Product8/1 -> Sqrt1/1
  Math Function4/1 -> Product8/1

== system simAttitudeControl/Controller/getRedAttRelatedPars/vectorNorm1 ==
  v : Inport
  Math Function4 : Math  Operator=transpose  SaturateOnIntegerOverflow=on
  Product8 : Product  Multiplication=Matrix(*)  RndMeth=Zero
  Sqrt1 : Sqrt  SaturateOnIntegerOverflow=on
  vNorm : Outport
  wires:
  Math Function4/1 -> Product8/1
  Product8/1 -> Sqrt1/1
  v/1 -> Math Function4/1, Product8/2
  Sqrt1/1 -> vNorm/1

== system simAttitudeControl/Controller/getRedAttRelatedPars/vectorNorm2 ==
  v : Inport
  Math Function4 : Math  Operator=transpose  SaturateOnIntegerOverflow=on
  Product8 : Product  Multiplication=Matrix(*)  RndMeth=Zero
  Sqrt1 : Sqrt  SaturateOnIntegerOverflow=on
  vNorm : Outport
  wires:
  Math Function4/1 -> Product8/1
  Product8/1 -> Sqrt1/1
  v/1 -> Math Function4/1, Product8/2
  Sqrt1/1 -> vNorm/1

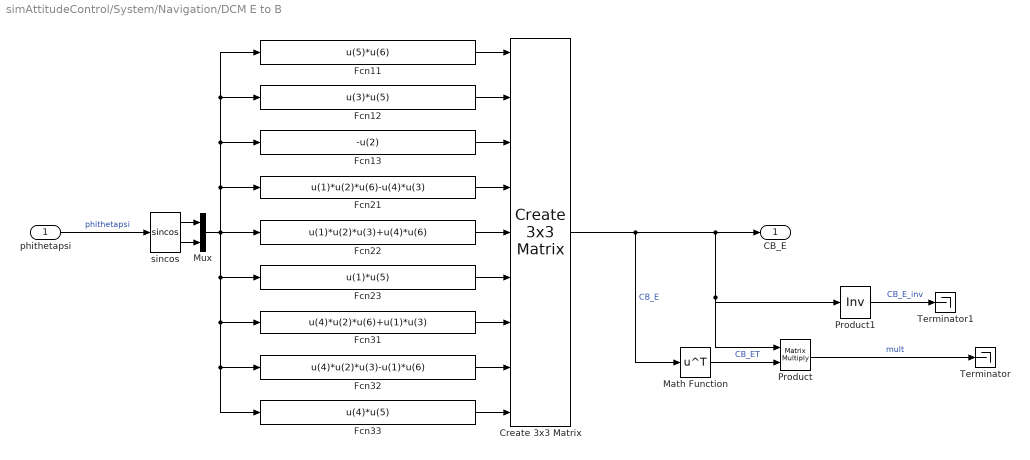
== system simAttitudeControl/System/Navigation/DCM E to B ==
  phithetapsi : Inport
  Create 3x3 Matrix : aerolibutil/Create 3x3 Matrix
  Fcn11 : Fcn  Expr=u(5)*u(6)
  Fcn12 : Fcn  Expr=u(3)*u(5)
  Fcn13 : Fcn  Expr=-u(2)
  Fcn21 : Fcn  Expr=u(1)*u(2)*u(6)-u(4)*u(3)
  Fcn22 : Fcn  Expr=u(1)*u(2)*u(3)+u(4)*u(6)
  Fcn23 : Fcn  Expr=u(1)*u(5)
  Fcn31 : Fcn  Expr=u(4)*u(2)*u(6)+u(1)*u(3)
  Fcn32 : Fcn  Expr=u(4)*u(2)*u(3)-u(1)*u(6)
  Fcn33 : Fcn  Expr=u(4)*u(5)
  Math Function : Math  Operator=transpose  SaturateOnIntegerOverflow=on
  Mux : Mux  Inputs=2
  Product : Product  Multiplication=Matrix(*)  RndMeth=Zero
  Product1 : Product  Inputs=/  Multiplication=Matrix(*)  RndMeth=Zero
  Terminator : Terminator
  Terminator1 : Terminator
  sincos : Trigonometry  Operator=sincos
  CB_E : Outport
  wires:
  sincos/1 -> Mux/1
  sincos/2 -> Mux/2
  Mux/1 -> Fcn32/1, Fcn33/1, Fcn31/1, Fcn23/1, Fcn22/1, Fcn11/1, Fcn12/1, Fcn13/1, Fcn21/1
  Fcn11/1 -> Create 3x3 Matrix/1
  Fcn12/1 -> Create 3x3 Matrix/2
  Fcn13/1 -> Create 3x3 Matrix/3
  Fcn21/1 -> Create 3x3 Matrix/4
  Fcn31/1 -> Create 3x3 Matrix/7
  Fcn22/1 -> Create 3x3 Matrix/5
  Fcn23/1 -> Create 3x3 Matrix/6
  Fcn32/1 -> Create 3x3 Matrix/8
  Fcn33/1 -> Create 3x3 Matrix/9
  phithetapsi/1 -> sincos/1  "phithetapsi"
  Create 3x3 Matrix/1 -> Math Function/1, CB_E/1, Product/1, Product1/1  "CB_E"
  Math Function/1 -> Product/2  "CB_ET"
  Product1/1 -> Terminator1/1  "CB_E_inv"
  Product/1 -> Terminator/1  "mult"

== system simAttitudeControl/getDist/calcParameters/DCM E to B1 ==
  phithetapsi : Inport
  Create 3x3 Matrix : aerolibutil/Create 3x3 Matrix
  Fcn11 : Fcn  Expr=u(5)*u(6)
  Fcn12 : Fcn  Expr=u(3)*u(5)
  Fcn13 : Fcn  Expr=-u(2)
  Fcn21 : Fcn  Expr=u(1)*u(2)*u(6)-u(4)*u(3)
  Fcn22 : Fcn  Expr=u(1)*u(2)*u(3)+u(4)*u(6)
  Fcn23 : Fcn  Expr=u(1)*u(5)
  Fcn31 : Fcn  Expr=u(4)*u(2)*u(6)+u(1)*u(3)
  Fcn32 : Fcn  Expr=u(4)*u(2)*u(3)-u(1)*u(6)
  Fcn33 : Fcn  Expr=u(4)*u(5)
  Mux : Mux  Inputs=2
  sincos : Trigonometry  Operator=sincos
  CB_E : Outport
  wires:
  Create 3x3 Matrix/1 -> CB_E/1  "CB_E"
  phithetapsi/1 -> sincos/1  "phithetapsi"
  Fcn33/1 -> Create 3x3 Matrix/9
  Fcn32/1 -> Create 3x3 Matrix/8
  Fcn23/1 -> Create 3x3 Matrix/6
  Fcn22/1 -> Create 3x3 Matrix/5
  Fcn31/1 -> Create 3x3 Matrix/7
  Fcn21/1 -> Create 3x3 Matrix/4
  Fcn13/1 -> Create 3x3 Matrix/3
  Fcn12/1 -> Create 3x3 Matrix/2
  Fcn11/1 -> Create 3x3 Matrix/1
  Mux/1 -> Fcn21/1, Fcn13/1, Fcn12/1, Fcn11/1, Fcn22/1, Fcn23/1, Fcn31/1, Fcn33/1, Fcn32/1
  sincos/2 -> Mux/2
  sincos/1 -> Mux/1

== system simAttitudeControl/getDist/getDistance/vectorNorm ==
  v : Inport
  Math Function4 : Math  Operator=transpose  SaturateOnIntegerOverflow=on
  Product8 : Product  Multiplication=Matrix(*)  RndMeth=Zero
  Sqrt1 : Sqrt  SaturateOnIntegerOverflow=on
  vNorm : Outport
  wires:
  Sqrt1/1 -> vNorm/1
  v/1 -> Product8/2, Math Function4/1
  Product8/1 -> Sqrt1/1
  Math Function4/1 -> Product8/1

== system simAttitudeControl/Controller/getRedAttRelatedPars/getDistance/vectorNorm ==
  v : Inport
  Math Function4 : Math  Operator=transpose  SaturateOnIntegerOverflow=on
  Product8 : Product  Multiplication=Matrix(*)  RndMeth=Zero
  Sqrt1 : Sqrt  SaturateOnIntegerOverflow=on
  vNorm : Outport
  wires:
  Sqrt1/1 -> vNorm/1
  v/1 -> Product8/2, Math Function4/1
  Product8/1 -> Sqrt1/1
  Math Function4/1 -> Product8/1
